simulink model "SIMULATION_7_C"  (Simulink 8.1)
settings: Solver=ode45  StartTime=0.0  StopTime=4  RelTol=1e-3
settings Model: Creator=prt01  LastModifiedBy=prt01
settings DebuggingCC: FcnCallInpInsideContextMsg=EnableAllAsWarning

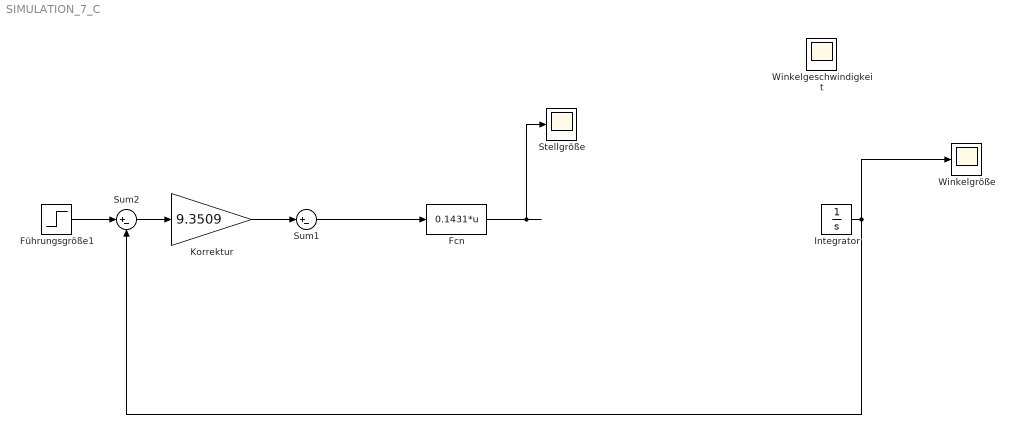
== system SIMULATION_7_C ==
  Fcn : Fcn  Expr=0.1431*u
  Führungsgröße1 : Step  After=90  SampleTime=0
  Integrator : Integrator
  Korrektur : Gain  Gain=9.3509
  Stellgröße : Scope
      settings: SaveName=ScopeData2
  Sum1 : Sum  Inputs=|+-
  Sum2 : Sum  Inputs=|+-
  Winkelgeschwindigkeit : Scope
  Winkelgröße : Scope
  wires:
  Führungsgröße1/1 -> Sum2/1
  Sum2/1 -> Korrektur/1
  Fcn/1 -> Stellgröße/1
  Korrektur/1 -> Sum1/1
  Sum1/1 -> Fcn/1
  ? -> Integrator/1, Sum1/2, Winkelgeschwindigkeit/1
  Integrator/1 -> Sum2/2, Winkelgröße/1
